simulink model "cannonball"  (R2021a)
settings: Solver=VariableStepAuto  StartTime=0.0  StopTime=5  RelTol=1e-3
libraries: simulink_extras x1, simulink x1
settings Model: Creator=jiaweichen  LastModifiedBy=jiaweichen

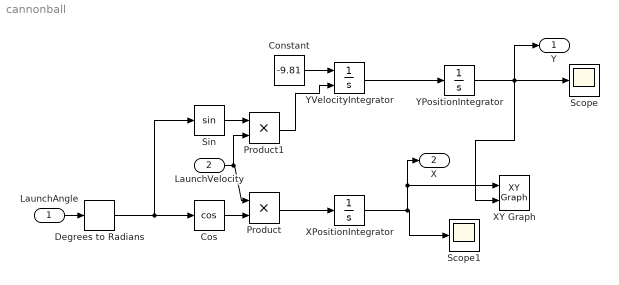
== system cannonball ==
  LaunchAngle : Inport
  LaunchVelocity : Inport  Port=2
  Constant : Constant  Value=-9.81
  Cos : Trigonometry  Operator=cos
  Degrees to Radians : simulink_extras/Transformations/Degrees to Radians
  Product : Product
  Product1 : Product
  Scope : Scope
  Scope1 : Scope
  Sin : Trigonometry
  XPositionIntegrator : Integrator
  XY Graph : simulink/Sinks/XY Graph  xmin=0  xmax=100  ymin=0  ymax=15  st=-1
  YPositionIntegrator : Integrator
  YVelocityIntegrator : Integrator  InitialConditionSource=external
  Y : Outport
  X : Outport  Port=2
  wires:
  Constant/1 -> YVelocityIntegrator/1
  YVelocityIntegrator/1 -> YPositionIntegrator/1
  LaunchVelocity/1 -> Product1/2, Product/1
  YPositionIntegrator/1 -> Y/1, XY Graph/2, Scope/1
  Degrees to Radians/1 -> Sin/1, Cos/1
  Sin/1 -> Product1/1
  Product1/1 -> YVelocityIntegrator/2
  Product/1 -> XPositionIntegrator/1
  Cos/1 -> Product/2
  XPositionIntegrator/1 -> X/1, XY Graph/1, Scope1/1
  LaunchAngle/1 -> Degrees to Radians/1
